simulink model "mpcACCsystem"  (R2023b)
settings: Solver=FixedStepAuto  StartTime=0.0  StopTime=simDuration  RelTol=1e-3
values from neighbouring files (symbols this model uses):
  ec_pos = 10    [mainACCcode.m]
  ec_vel = 20    [mainACCcode.m]    (also in plotACC.m = logsout.getElement('ec_vel'))
  lc_pos = 50    [mainACCcode.m]
  lc_vel = 25    [mainACCcode.m]    (also in plotACC.m = logsout.getElement('lc_vel'))
  setVel = evalin('base', 'setVel')    [mainACCcode.m]
  timeGap = evalin('base', 'timeGap')    [mainACCcode.m]
  Ts = 0.1    [mainACCcode.m]    (also in setUpACCWorkspaceVars.m)
libraries: mpcadaslib x1
settings Model: Creator=The MathWorks, Inc.  LastModifiedBy=Subhadeep Das
settings SolverCC: AlgebraicLoopSolver=TrustRegion
settings DataIOCC: ReturnWorkspaceOutputs=off
settings DebuggingCC: UnconnectedInputMsg=warning  UnconnectedOutputMsg=warning  UnconnectedLineMsg=warning  ArithmeticOperatorsInVariantConditions=warning
settings ModelReferenceCC: EnableRefExpFcnMdlSchedulingChecks=on
settings SFSimCC: SimUseLocalCustomCode=off  CustomCodeUndefinedFunction=UseInterfaceOnly
settings RTWCC: RTWUseLocalCustomCode=off
settings CodeAppCC: StateflowObjectComments=on

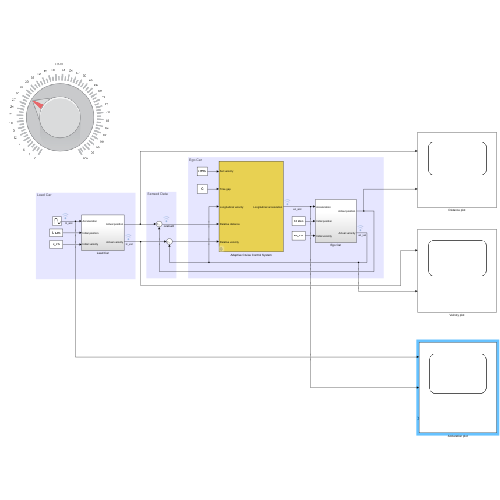
[thumbnail: Simulink's stored preview of the top-level diagram]
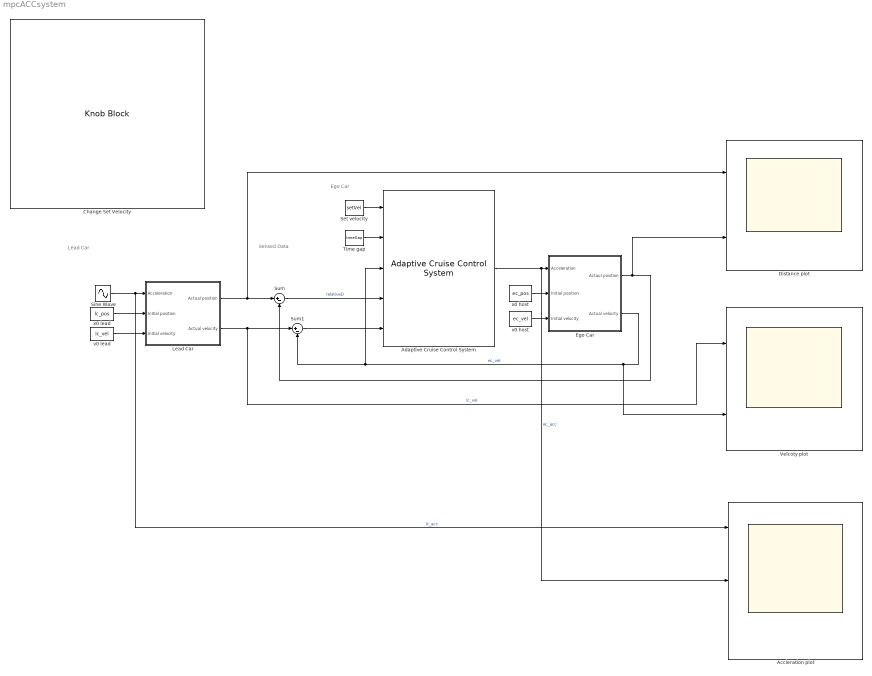
== system mpcACCsystem ==
  note: Sensed Data
  note: Lead Car
  note: Ego Car
  Accleration plot : Scope  NumInputPorts=3
  Adaptive Cruise Control System : mpcadaslib/Adaptive Cruise Control System  EgoModel=tf(1,[0.5,1,0])  InitialEgoVelocity=20  DefaultSpacing=10  MaxVelocity=50  MinAcceleration=-3  amin_ext=off  MaxAcceleration=2  amax_ext=off  Ts=0.1  PredictionHorizon=30  ControllerBehavior=0.5  suboptimal=off  maxiter=10  datatypeopt=double  optmode=off  trackmode=off
  Change Set Velocity : KnobBlock
  Distance plot : Scope  NumInputPorts=2
  Ego Car : Subsystem
  Lead Car : Subsystem
  Set velocity : Constant  Value=setVel  SampleTime=Ts
  Sine Wave : Sin  Amplitude=0.6  Frequency=0.2  SampleTime=Ts
  Sum : Sum  Inputs=|+-
  Sum1 : Sum  Inputs=|+-
  Time gap : Constant  Value=timeGap  SampleTime=Ts
  Velcoty plot : Scope  NumInputPorts=2
  v0 host : Constant  Value=ec_vel  SampleTime=Ts
  v0 lead : Constant  Value=lc_vel  SampleTime=Ts
  x0 host : Constant  Value=ec_pos  SampleTime=Ts
  x0 lead : Constant  Value=lc_pos  SampleTime=Ts
  wires:
  x0 lead/1 -> Lead Car/2(Initial position)
  v0 lead/1 -> Lead Car/3(Initial velocity)
  x0 host/1 -> Ego Car/2(Initial position)
  Ego Car/1(Actaul position) -> Distance plot/2, Sum/2
  Ego Car/2(Actual velocity) -> Velcoty plot/2, Adaptive Cruise Control System/3, Sum1/2  "ec_vel"
  v0 host/1 -> Ego Car/3(Initial velocity)
  Set velocity/1 -> Adaptive Cruise Control System/1
  Adaptive Cruise Control System/1 -> Accleration plot/2, Ego Car/1(Acceleration)  "ec_acc"
  Lead Car/1(Actual position) -> Distance plot/1, Sum/1
  Sum1/1 -> Adaptive Cruise Control System/5
  Time gap/1 -> Adaptive Cruise Control System/2
  Sine Wave/1 -> Accleration plot/1, Lead Car/1(Acceleration)  "lc_acc"
  Lead Car/2(Actual velocity) -> Velcoty plot/1, Sum1/1  "lc_vel"
  Sum/1 -> Adaptive Cruise Control System/4  "relativeD"

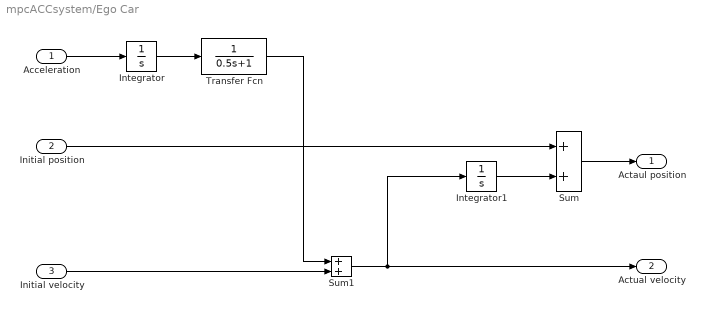
== system mpcACCsystem/Ego Car ==
  Acceleration : Inport
  Initial position : Inport  Port=2
  Initial velocity : Inport  Port=3
  Integrator : Integrator
  Integrator1 : Integrator
  Sum : Sum
  Sum1 : Sum
  Transfer Fcn : TransferFcn  Denominator=[0.5 1]
  Actaul position : Outport  VectorParamsAs1DForOutWhenUnconnected=off
  Actual velocity : Outport  Port=2  VectorParamsAs1DForOutWhenUnconnected=off
  wires:
  Sum1/1 -> Integrator1/1, Actual velocity/1
  Initial velocity/1 -> Sum1/2
  Sum/1 -> Actaul position/1
  Transfer Fcn/1 -> Sum1/1
  Integrator/1 -> Transfer Fcn/1
  Acceleration/1 -> Integrator/1
  Initial position/1 -> Sum/1
  Integrator1/1 -> Sum/2

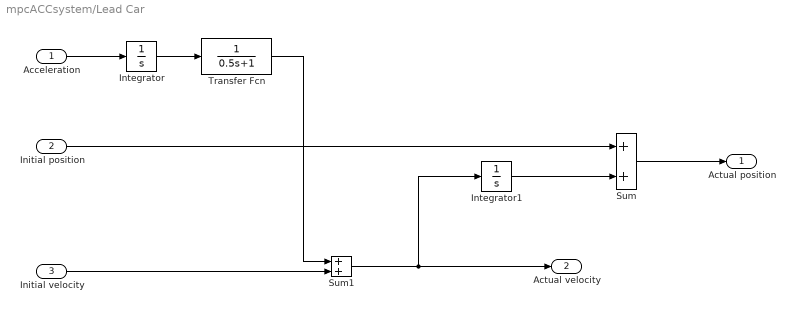
== system mpcACCsystem/Lead Car ==
  Acceleration : Inport
  Initial position : Inport  Port=2
  Initial velocity : Inport  Port=3
  Integrator : Integrator
  Integrator1 : Integrator
  Sum : Sum
  Sum1 : Sum
  Transfer Fcn : TransferFcn  Denominator=[0.5 1]
  Actual position : Outport  VectorParamsAs1DForOutWhenUnconnected=off
  Actual velocity : Outport  Port=2  VectorParamsAs1DForOutWhenUnconnected=off
  wires:
  Transfer Fcn/1 -> Sum1/1
  Initial velocity/1 -> Sum1/2
  Sum/1 -> Actual position/1
  Integrator/1 -> Transfer Fcn/1
  Sum1/1 -> Integrator1/1, Actual velocity/1
  Acceleration/1 -> Integrator/1
  Initial position/1 -> Sum/1
  Integrator1/1 -> Sum/2
